simulink model "platoon1"  (R2023a)
settings: Solver=ode2  StartTime=0.0  StopTime=20  FixedStep=1/600  RelTol=1e-3  EnableMultiTasking=on
undefined symbols (not defined in the file or in its folder): HIL, qc_get_step_size
libraries: simulink x29, quarc_library x29, slpidlib x27, cstblocks x23, eeStairGenerator x1
(part 1 of 4)
settings Model: ExtModeTrigDuration=10000  Creator=ritvi  LastModifiedBy=ritvi
settings SolverCC: AlgebraicLoopSolver=TrustRegion  PositivePriorityOrder=on
settings DataIOCC: ReturnWorkspaceOutputs=off
settings DebuggingCC: UnconnectedInputMsg=warning  UnconnectedOutputMsg=warning  UnconnectedLineMsg=warning  ArithmeticOperatorsInVariantConditions=warning
settings HardwareCC: ProdBitPerLong=64  ProdLargestAtomicInteger=LongLong  ProdLargestAtomicFloat=Double  ProdLongLongMode=on  ProdHWDeviceType=ARM Compatible->ARM 64-bit (LP64)
settings ModelReferenceCC: EnableRefExpFcnMdlSchedulingChecks=on
settings SFSimCC: SimUseLocalCustomCode=off  CustomCodeUndefinedFunction=UseInterfaceOnly
settings RTWCC: Description=QUARC Linux Nvidia Target (QCar) Using Toolchain  SystemTargetFile=quarc_linux_nvidia.tlc  TemplateMakefile=quarc_default_tmf  RTWUseLocalCustomCode=off  Toolchain=QUARC linux_nvidia | gmake (64-bit Windows)  BuildConfiguration=Faster Runs
settings CodeAppCC: StateflowObjectComments=on
settings STFCustomTargetCC: SystemTargetFile=quarc_linux_nvidia.tlc
settings GRTTargetCC: ParMdlRefBuildCompliant=off  CompOptLevelCompliant=off  CombineOutputUpdateFcns=off  MatFileLogging=off  CPPClassGenCompliant=off  GRTInterface=on  ExtMode=on  ExtModeMexFile=quarc_comm  ExtModeMexArgs='-w -d /tmp -uri %u', 'tcpip://192.168.1.9'
settings ConfigComp: CovMetricSettings=dswe

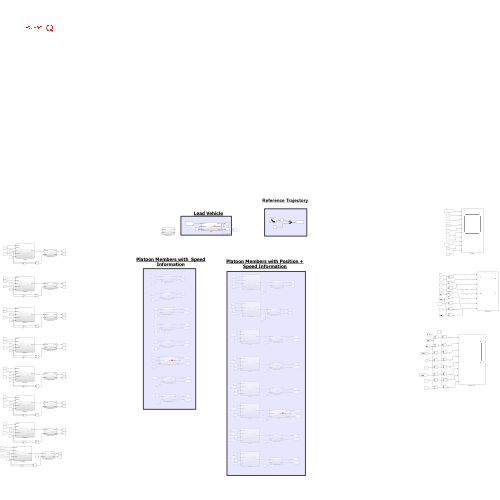
[thumbnail: Simulink's stored preview of the top-level diagram]
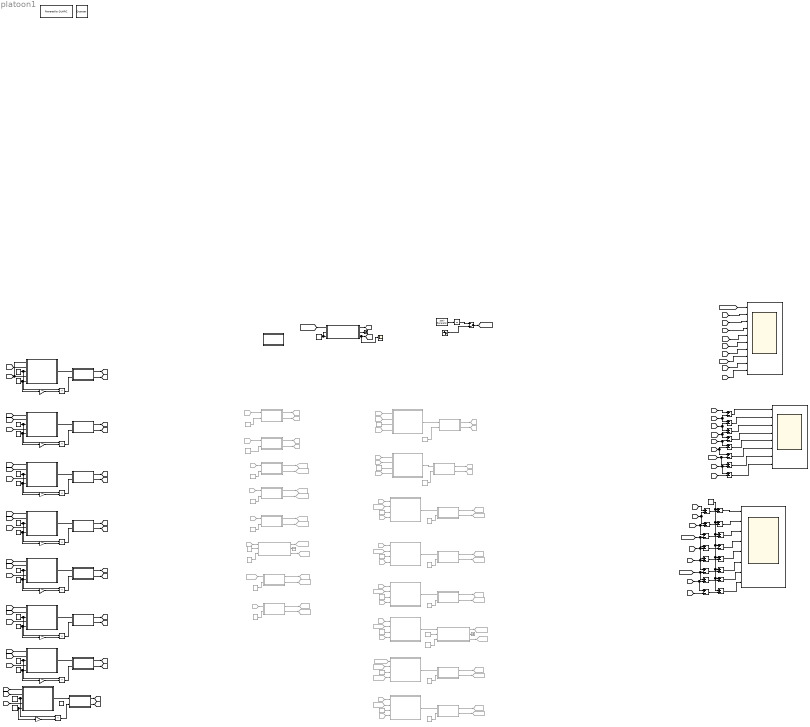
== system platoon1 ==
  note: Platoon Members with Speed Information
  note: Lead Vehicle
  note: Reference Trajectory
  note: Platoon Members with Position + Speed Information
  Add{,1..23} (24 alike) : Sum  Inputs=+-
  Constant : Constant  Value=0
  Constant1 : Constant  Commented=on  Value=0
  Constant{3,6..7,9..10,12,15,18} (8 alike) : Constant  Commented=on  Value=0.5
  Constant11 : Constant  Commented=on  Value=-3.5
  Constant13 : Constant  Commented=on  Value=-4
  Constant{14,19,23,26,28,30,36,40,43} (9 alike) : Constant  Value=0.5
  Constant16 : Constant  Commented=on  Value=-0.5
  Constant17 : Constant
  Constant2 : Constant  Commented=on  Value=-2
  Constant20 : Constant  Commented=on  Value=-1
  Constant21 : Constant  Value=2
  Constant22 : Constant  Commented=on  Value=0
  Constant24 : Constant  Value=3
  Constant25 : Constant  Commented=on  Value=-3.5
  Constant27 : Constant  Value=4
  Constant29 : Constant  Commented=on  Value=-4
  Constant31 : Constant  Value=5
  Constant32 : Constant  Commented=on  Value=-0.5
  Constant33 : Constant  Value=6
  Constant34 : Constant  Commented=on  Value=-2
  Constant35 : Constant  Commented=on  Value=-1
  Constant37 : Constant  Commented=on  Value=-2.5
  Constant38 : Constant  Commented=on  Value=-3
  Constant39 : Constant  Value=7
  Constant4 : Constant  Commented=on  Value=-2.5
  Constant41 : Constant  Commented=on  Value=-1.5
  Constant42 : Constant  Value=8
  Constant44 : Constant  Value=0
  Constant5 : Constant  Commented=on  Value=-3
  Constant8 : Constant  Commented=on  Value=-1.5
  Controller : Subsystem  Commented=on
  Controller1 : Subsystem  Commented=on
  Controller10 : Subsystem
  Controller11 : Subsystem
  Controller12 : Subsystem
  Controller13 : Subsystem
  Controller14 : Subsystem
  Controller15 : Subsystem
  Controller2 : Subsystem  Commented=on
  Controller3 : Subsystem  Commented=on
  Controller4 : Subsystem  Commented=on
  Controller5 : Subsystem  Commented=on
  Controller6 : Subsystem  Commented=on
  Controller7 : Subsystem  Commented=on
  Controller8 : Subsystem
  Controller9 : Subsystem
  Distance errors : Scope  NumInputPorts=8
  From : From  Commented=on  GotoTag=pos1
  From1 : From  Commented=on  GotoTag=pos0
  From10 : From  Commented=on  GotoTag=pos5
  From11 : From  Commented=on  GotoTag=vel4
  From12 : From  Commented=on  GotoTag=pos4
  From13 : From  Commented=on  GotoTag=pos7
  From2 : From  Commented=on  GotoTag=pos2
  From23 : From  Commented=on  GotoTag=vel0
  From24 : From  Commented=on  GotoTag=vel1
  From27 : From  Commented=on  GotoTag=vel6_QCar
  From28 : From  Commented=on  GotoTag=pos6_QCar
  From3 : From  Commented=on  GotoTag=pos1
  From4 : From  Commented=on  GotoTag=pos6_QCar
  From41 : From  Commented=on  GotoTag=pos8
  From42 : From  Commented=on  GotoTag=vel7
  From43 : From  Commented=on  GotoTag=pos7
  From47 : From  Commented=on  GotoTag=pos4
  From48 : From  Commented=on  GotoTag=vel3
  From49 : From  Commented=on  GotoTag=pos3
  From5 : From  Commented=on  GotoTag=vel5
  From6 : From  Commented=on  GotoTag=pos5
  From60 : From  Commented=on  GotoTag=vel4
  From66 : From  Commented=on  GotoTag=vel0
  From68 : From  Commented=on  GotoTag=vel1
  From69 : From  Commented=on  GotoTag=vel6_QCar
  From7 : From  Commented=on  GotoTag=pos3
  From74 : From  Commented=on  GotoTag=vel7
  From77 : From  Commented=on  GotoTag=vel3
  From79 : From  Commented=on  GotoTag=vel5
  From8 : From  Commented=on  GotoTag=vel2
  From82 : From  Commented=on  GotoTag=vel2
  From9 : From  Commented=on  GotoTag=pos2
  Gain{1..8} (8 alike) : Gain  Gain=-1
  Goto10 : Goto  Commented=on  GotoTag=vel2
  Goto11 : Goto  Commented=on  GotoTag=vel6_QCar
  Goto12 : Goto  Commented=on  GotoTag=pos5
  Goto13 : Goto  Commented=on  GotoTag=vel7
  Goto14 : Goto  Commented=on  GotoTag=pos7
  Goto15 : Goto  Commented=on  GotoTag=vel8
  Goto16 : Goto  Commented=on  GotoTag=pos8
  Goto2 : Goto  Commented=on  GotoTag=vel3
  Goto3 : Goto  Commented=on  GotoTag=pos1
  Goto31 : Goto  Commented=on  GotoTag=vel1
  Goto33 : Goto  Commented=on  GotoTag=vel2
  Goto34 : Goto  Commented=on  GotoTag=vel6_QCar
  Goto35 : Goto  Commented=on  GotoTag=pos5
  Goto36 : Goto  Commented=on  GotoTag=vel7
  Goto37 : Goto  Commented=on  GotoTag=pos7
  Goto38 : Goto  Commented=on  GotoTag=vel8
  Goto39 : Goto  Commented=on  GotoTag=pos8
  Goto4 : Goto  Commented=on  GotoTag=pos6_QCar
  Goto40 : Goto  Commented=on  GotoTag=vel3
  Goto41 : Goto  Commented=on  GotoTag=pos1
  Goto42 : Goto  Commented=on  GotoTag=vel1
  Goto43 : Goto  Commented=on  GotoTag=pos6_QCar
  Goto44 : Goto  Commented=on  GotoTag=pos2
  Goto45 : Goto  Commented=on  GotoTag=pos3
  Goto46 : Goto  Commented=on  GotoTag=vel4
  Goto47 : Goto  Commented=on  GotoTag=pos4
  Goto48 : Goto  Commented=on  GotoTag=vel5
  Goto5 : Goto  Commented=on  GotoTag=pos2
  Goto6 : Goto  Commented=on  GotoTag=pos3
  Goto7 : Goto  Commented=on  GotoTag=vel4
  Goto8 : Goto  Commented=on  GotoTag=pos4
  Goto9 : Goto  Commented=on  GotoTag=vel5
  Integrator2 : Integrator
  Manual Switch : ManualSwitch  CurrentSetting=0
  Powered by QUARC : quarc_library/Logos/Powered by QUARC
  Product{,1..7} (8 alike) : Product
  QCar1 : Subsystem  Commented=on
  QCar2 : Subsystem  Commented=on
  QCar4 : Subsystem
  Quanser : quarc_library/Logos/Quanser
  Scope : Scope
  Sine Wave : Sin  Amplitude=0.4  Frequency=0.5  SampleTime=qc_get_step_size
  Stair Generator : eeStairGenerator/Stair Generator  LabelModeActiveChoice=Discrete  TimeInput=[5 7 9 13 15 17]  AmplitudeInput=[0.1 0.15 0 -0.1 -0.15 0]  SampleTime=1/600  RepeatPattern=off  OutDataTypeStr=double
      settings: LibrarySourceBlock=ee_sl_lib/General Control/Stair Generator
  Terminator : Terminator
  Terminator1 : Terminator  Commented=on
  Terminator2 : Terminator  Commented=on
  Velocities : Scope  NumInputPorts=10
  Velocity errors : Scope  NumInputPorts=8
  Virtual Car (TF) : Subsystem
  Virtual Car (TF)1 : Subsystem  Commented=on
  Virtual Car (TF)10 : Subsystem
  Virtual Car (TF)11 : Subsystem
  Virtual Car (TF)12 : Subsystem
  Virtual Car (TF)13 : Subsystem
  Virtual Car (TF)14 : Subsystem
  Virtual Car (TF)15 : Subsystem
  Virtual Car (TF)16 : Subsystem  Commented=on
  Virtual Car (TF)17 : Subsystem  Commented=on
  Virtual Car (TF)18 : Subsystem  Commented=on
  Virtual Car (TF)19 : Subsystem  Commented=on
  Virtual Car (TF)2 : Subsystem  Commented=on
  Virtual Car (TF)20 : Subsystem  Commented=on
  Virtual Car (TF)21 : Subsystem  Commented=on
  Virtual Car (TF)22 : Subsystem
  Virtual Car (TF)3 : Subsystem  Commented=on
  Virtual Car (TF)4 : Subsystem  Commented=on
  Virtual Car (TF)5 : Subsystem  Commented=on
  Virtual Car (TF)6 : Subsystem  Commented=on
  Virtual Car (TF)7 : Subsystem  Commented=on
  Virtual Car (TF)8 : Subsystem  Commented=on
  Virtual Car (TF)9 : Subsystem
  wires:
  QCar1/1(ActSpeed) -> Goto11/1  "v6_Q"
  QCar1/2(ActHeading) -> Terminator1/1
  QCar1/3(position) -> Goto4/1  "p6_Q"
  Controller2/1(Speed) -> QCar1/1(RefSpeed)
  Constant1/1 -> QCar1/2(RefHeading)
  Constant5/1 -> QCar1/3(InitPos)
  From6/1 -> Controller2/1(PosLead)
  From4/1 -> Controller2/2(PosEgo)
  Constant6/1 -> Controller2/3(d_ref)
  From5/1 -> Controller2/4(VelLead)
  Virtual Car (TF)4/1(position) -> Goto8/1  "p4"
  From47/1 -> Controller4/2(PosEgo)
  Add13/1 -> Distance errors/6  "de6"
  Controller1/1(Speed) -> Virtual Car (TF)2/1(RefSpeed)
  Constant8/1 -> Virtual Car (TF)3/2(InitPos)
  [pos1] -> Add18/1, Add6/2
  Controller3/1(Speed) -> Virtual Car (TF)3/1(RefSpeed)
  Constant16/1 -> Virtual Car (TF)1/2(InitPos)
  Virtual Car (TF)1/1(position) -> Goto3/1  "p1"
  Add8/1 -> Add9/2
  [vel3] -> Add2/2, Add3/1
  Add2/1 -> Velocity errors/3  "ve3"
  [vel5] -> Velocities/7
  Virtual Car (TF)3/2(speed) -> Goto2/1  "v3"
  Virtual Car (TF)2/2(speed) -> Goto10/1  "v2"
  Constant20/1 -> Virtual Car (TF)2/2(InitPos)
  QCar4/3(position) -> Scope/1, [pos0]  "p0"
  Virtual Car (TF)1/2(speed) -> Goto31/1  "v1"
  Virtual Car (TF)2/1(position) -> Goto5/1  "p2"
  [vel0] -> Add/1
  [vel0] -> Velocities/2
  [vel1] -> Add/2, Add1/1
  From24/1 -> Controller1/4(VelLead)
  Add3/1 -> Velocity errors/4  "ve4"
  Add6/1 -> Add7/2
  Add5/1 -> Velocity errors/5  "ve5"
  [pos4] -> Add10/1, Add8/2
  Controller/1(Speed) -> Virtual Car (TF)1/1(RefSpeed)
  QCar4/1(ActSpeed) -> [vel0]  "v0"
  Add17/1 -> Distance errors/3  "de3"
  Add1/1 -> Velocity errors/2  "ve2"
  Add16/1 -> Add17/2
  [pos0] -> Add6/1
  Add/1 -> Velocity errors/1  "ve1"
  [pos5] -> Add12/1, Add10/2
  Constant14/1 -> Add7/1, Add19/1, Add17/1, Add9/1, Add11/1, Add23/1, Add20/1, Add13/1
  Add12/1 -> Add13/2
  Add19/1 -> Distance errors/2  "de2"
  Add9/1 -> Distance errors/4  "de4"
  [pos6] -> Add15/1, Add12/2
  Constant2/1 -> Virtual Car (TF)4/2(InitPos)
  Constant3/1 -> Controller4/3(d_ref)
  From48/1 -> Controller4/4(VelLead)
  From13/1 -> Controller6/2(PosEgo)
  From11/1 -> Controller5/4(VelLead)
  [vel6] -> Add14/1, Add4/2
  Controller4/1(Speed) -> Virtual Car (TF)4/1(RefSpeed)
  Constant18/1 -> Controller/3(d_ref)
  Add14/1 -> Velocity errors/7  "ve7"
  From28/1 -> Controller6/1(PosLead)
  Add20/1 -> Distance errors/7  "de7"
  [pos7] -> Add22/1, Add15/2
  From8/1 -> Controller3/4(VelLead)
  Add4/1 -> Velocity errors/6  "ve6"
  [LeadRefSpeed] -> QCar4/1(RefSpeed)
  Controller5/1(Speed) -> Virtual Car (TF)5/1(RefSpeed)
  Virtual Car (TF)3/1(position) -> Goto6/1  "p3"
  Controller6/1(Speed) -> Virtual Car (TF)6/1(RefSpeed)
  From42/1 -> Controller7/4(VelLead)
  Virtual Car (TF)4/2(speed) -> Goto7/1  "v4"
  [vel4] -> Velocities/6
  Virtual Car (TF)6/1(position) -> Goto14/1  "p7"
  Constant4/1 -> Virtual Car (TF)5/2(InitPos)
  [vel7] -> Velocities/9
  Controller7/1(Speed) -> Virtual Car (TF)7/1(RefSpeed)
  From3/1 -> Controller1/1(PosLead)
  [vel2] -> Velocities/4
  [vel3] -> Velocities/5
  From27/1 -> Controller6/4(VelLead)
  From12/1 -> Controller5/1(PosLead)
  Add18/1 -> Add19/2
  Virtual Car (TF)6/2(speed) -> Goto13/1  "v7"
  Virtual Car (TF)5/2(speed) -> Goto9/1  "v5"
  [vel2] -> Add1/2, Add2/1
  From/1 -> Controller/2(PosEgo)
  [pos3] -> Add8/1, Add16/2
  [LeadRefSpeed] -> Velocities/1
  From10/1 -> Controller5/2(PosEgo)
  [vel6] -> Velocities/8
  Constant7/1 -> Controller5/3(d_ref)
  Constant15/1 -> Controller7/3(d_ref)
  Constant/1 -> QCar4/2(RefHeading), QCar4/3(InitPos)
  Add11/1 -> Distance errors/5  "de5"
  From41/1 -> Controller7/2(PosEgo)
  From2/1 -> Controller1/2(PosEgo)
  From9/1 -> Controller3/1(PosLead)
  Constant11/1 -> Virtual Car (TF)6/2(InitPos)
  Add10/1 -> Add11/2
  From7/1 -> Controller3/2(PosEgo)
  Constant9/1 -> Controller3/3(d_ref)
  Add7/1 -> Distance errors/1  "de1"
  Constant12/1 -> Controller6/3(d_ref)
  Virtual Car (TF)7/1(position) -> Goto16/1  "p8"
  [vel1] -> Velocities/3
  [vel5] -> Add4/1, Add5/2
  Constant13/1 -> Virtual Car (TF)7/2(InitPos)
  [vel4] -> Add3/2, Add5/1
  From1/1 -> Controller/1(PosLead)
  Virtual Car (TF)5/1(position) -> Goto12/1  "p5"
  Virtual Car (TF)7/2(speed) -> Goto15/1  "v8"
  [pos2] -> Add16/1, Add18/2
  [vel7] -> Add21/1, Add14/2
  Constant10/1 -> Controller1/3(d_ref)
  From43/1 -> Controller7/1(PosLead)
  Add15/1 -> Add20/2
  From49/1 -> Controller4/1(PosLead)
  From23/1 -> Controller/4(VelLead)
  [vel8] -> Velocities/10
  [vel8] -> Add21/2
  Add21/1 -> Velocity errors/8  "ve8"
  Add22/1 -> Add23/2
  [pos8] -> Add22/2
  Add23/1 -> Distance errors/8  "de8"
  Virtual Car (TF)19/1(position) -> Goto35/1  "p5"
  Virtual Car (TF)21/2(speed) -> Goto38/1  "v8"
  From69/1 -> Virtual Car (TF)20/1(RefSpeed)
  Virtual Car (TF)19/2(speed) -> Goto48/1  "v5"
  Virtual Car (TF)20/2(speed) -> Goto36/1  "v7"
  Virtual Car (TF)17/1(position) -> Goto45/1  "p3"
  Virtual Car (TF)18/2(speed) -> Goto46/1  "v4"
  From74/1 -> Virtual Car (TF)21/1(RefSpeed)
  From82/1 -> Virtual Car (TF)17/1(RefSpeed)
  Virtual Car (TF)20/1(position) -> Goto37/1  "p7"
  From60/1 -> Virtual Car (TF)19/1(RefSpeed)
  Constant34/1 -> Virtual Car (TF)18/2(InitPos)
  Virtual Car (TF)16/1(position) -> Goto44/1  "p2"
  Constant35/1 -> Virtual Car (TF)16/2(InitPos)
  Virtual Car (TF)21/1(position) -> Goto39/1  "p8"
  Virtual Car (TF)17/2(speed) -> Goto40/1  "v3"
  Virtual Car (TF)16/2(speed) -> Goto33/1  "v2"
  Constant32/1 -> Virtual Car (TF)8/2(InitPos)
  Constant37/1 -> Virtual Car (TF)19/2(InitPos)
  Constant25/1 -> Virtual Car (TF)20/2(InitPos)
  Virtual Car (TF)8/1(position) -> Goto41/1  "p1"
  Constant41/1 -> Virtual Car (TF)17/2(InitPos)
  From66/1 -> Virtual Car (TF)8/1(RefSpeed)
  Virtual Car (TF)18/1(position) -> Goto47/1  "p4"
  From77/1 -> Virtual Car (TF)18/1(RefSpeed)
  Virtual Car (TF)8/2(speed) -> Goto42/1  "v1"
  From79/1 -> QCar2/1(RefSpeed)
  Constant29/1 -> Virtual Car (TF)21/2(InitPos)
  QCar2/2(ActHeading) -> Terminator2/1
  QCar2/1(ActSpeed) -> Goto34/1  "v6_Q"
  Constant38/1 -> QCar2/3(InitPos)
  QCar2/3(position) -> Goto43/1  "p6_Q"
  Constant22/1 -> QCar2/2(RefHeading)
  From68/1 -> Virtual Car (TF)16/1(RefSpeed)
  [pos0] -> Controller13/4(PosLead)
  Virtual Car (TF)14/1(position) -> [pos7]  "p7"
  Product6/1 -> Virtual Car (TF)14/2(InitPos)
  Gain7/1 -> Product6/2
  Controller13/1(Speed) -> Virtual Car (TF)14/1(RefSpeed)
  [pos6] -> Controller13/1(PosPred)
  Constant40/1 -> Product6/1, Controller13/3(d_ref)
  Constant39/1 -> Controller13/5(i), Gain7/1
  [pos4] -> Controller11/1(PosPred)
  Constant31/1 -> Controller11/5(i), Gain5/1
  Virtual Car (TF)12/2(speed) -> [vel5]  "v5"
  Constant30/1 -> Product4/1, Controller11/3(d_ref)
  [pos0] -> Controller11/4(PosLead)
  Gain5/1 -> Product4/2
  Product4/1 -> Virtual Car (TF)12/2(InitPos)
  [pos5] -> Controller11/2(PosEgo)
  Controller11/1(Speed) -> Virtual Car (TF)12/1(RefSpeed)
  Constant33/1 -> Controller12/5(i), Gain6/1
  Gain6/1 -> Product5/2
  [pos6] -> Controller12/2(PosEgo)
  Controller12/1(Speed) -> Virtual Car (TF)13/1(RefSpeed)
  Virtual Car (TF)13/1(position) -> [pos6]  "p6"
  Product1/1 -> Virtual Car (TF)9/2(InitPos)
  [pos2] -> Controller9/2(PosEgo)
  Virtual Car (TF)9/1(position) -> [pos2]  "p2"
  Controller9/1(Speed) -> Virtual Car (TF)9/1(RefSpeed)
  Constant23/1 -> Product1/1, Controller9/3(d_ref)
  [pos0] -> Controller9/4(PosLead)
  Virtual Car (TF)14/2(speed) -> [vel7]  "v7"
  [pos1] -> Controller8/2(PosEgo)
  [pos7] -> Controller13/2(PosEgo)
  [pos0] -> Controller8/1(PosPred), Controller8/4(PosLead)
  [pos5] -> Controller12/1(PosPred)
  Constant28/1 -> Product3/1, Controller10/3(d_ref)
  Virtual Car (TF)11/2(speed) -> [vel4]  "v4"
  Gain2/1 -> Product1/2
  [pos0] -> Controller10/4(PosLead)
  Constant27/1 -> Controller10/5(i), Gain4/1
  Product3/1 -> Virtual Car (TF)11/2(InitPos)
  Virtual Car (TF)15/2(speed) -> [vel1]  "v1"
  [pos0] -> Controller12/4(PosLead)
  Gain4/1 -> Product3/2
  Gain1/1 -> Product/2
  [pos3] -> Controller10/1(PosPred)
  Constant19/1 -> Product/1, Controller8/3(d_ref)
  Product5/1 -> Virtual Car (TF)13/2(InitPos)
  Controller8/1(Speed) -> Virtual Car (TF)15/1(RefSpeed)
  Virtual Car (TF)15/1(position) -> [pos1]  "p1"
  Virtual Car (TF)12/1(position) -> [pos5]  "p5"
  Constant26/1 -> Product2/1, Controller14/3(d_ref)
  Virtual Car (TF)10/2(speed) -> [vel3]  "v3"
  [pos0] -> Controller14/4(PosLead)
  Constant24/1 -> Controller14/5(i), Gain3/1
  [pos2] -> Controller14/1(PosPred)
  Virtual Car (TF)13/2(speed) -> [vel6]  "v6"
  Constant21/1 -> Controller9/5(i), Gain2/1
  Gain3/1 -> Product2/2
  Constant36/1 -> Product5/1, Controller12/3(d_ref)
  Product2/1 -> Virtual Car (TF)10/2(InitPos)
  Virtual Car (TF)10/1(position) -> [pos3]  "p3"
  Constant17/1 -> Controller8/5(i), Gain1/1
  Controller10/1(Speed) -> Virtual Car (TF)11/1(RefSpeed)
  Controller14/1(Speed) -> Virtual Car (TF)10/1(RefSpeed)
  Virtual Car (TF)11/1(position) -> [pos4]  "p4"
  [pos1] -> Controller9/1(PosPred)
  [pos4] -> Controller10/2(PosEgo)
  Virtual Car (TF)9/2(speed) -> [vel2]  "v2"
  [pos3] -> Controller14/2(PosEgo)
  Product/1 -> Virtual Car (TF)15/2(InitPos)
  [pos8] -> Controller15/2(PosEgo)
  [pos0] -> Controller15/4(PosLead)
  Product7/1 -> Virtual Car (TF)22/2(InitPos)
  Controller15/1(Speed) -> Virtual Car (TF)22/1(RefSpeed)
  Constant42/1 -> Controller15/5(i), Gain8/1
  Gain8/1 -> Product7/2
  Constant43/1 -> Product7/1, Controller15/3(d_ref)
  [pos7] -> Controller15/1(PosPred)
  Virtual Car (TF)22/2(speed) -> [vel8]  "v8"
  Virtual Car (TF)22/1(position) -> [pos8]  "p8"
  Integrator2/1 -> Manual Switch/1
  Stair Generator/1 -> Integrator2/1
  Sine Wave/1 -> Manual Switch/2
  Manual Switch/1 -> [LeadRefSpeed]  "v_ref"
  QCar4/2(ActHeading) -> Terminator/1

== system platoon1/Controller ==
  PosLead : Inport
  PosEgo : Inport  Port=2
  d_ref : Inport  Port=3
  VelLead : Inport  Port=4
  Add : Sum  Inputs=+-
  Add1 : Sum  Inputs=+-
  Add2 : Sum  Inputs=+-
  Discrete Derivative : simulink/Discrete/Discrete Derivative  Commented=on  gainval=1.0  ICPrevScaledInput=0.0  OutMin=[]  OutMax=[]  OutDataType=fixdt(1, 16)  OutScaling=2^-10  DoSatur=off
  Integrator : Integrator  Commented=on
  Kd : Gain  Commented=on
  Ki : Gain  Commented=on
  Kp : Gain  Commented=on
  PID Controller : slpidlib/PID Controller  Controller=PID  Form=Parallel  TimeDomain=Continuous-time  UseExternalTs=off  SampleTime=-1  IntegratorMethod=Forward Euler  FilterMethod=Forward Euler  ControllerParametersSource=internal  P=3.40490772994016  I=1.59625421797035  UseKiTs=off  D=0.569076840427193  N=614.736952919996  UseFilter=on  TunerSelectOption=Transfer Function Based (PID Tuner App)  InitialConditionSource=internal  InitialConditionForIntegrator=0  InitialConditionForFilter=0  DifferentiatorICPrevScaledInput=0  ExternalReset=none  TrackingMode=off  Kt=1  LimitOutput=off  SatLimitsSource=internal  UpperSaturationLimit=inf  LowerSaturationLimit=-inf  LinearizeAsGain=on  AntiWindupMode=none  Kb=1  LimitIntegrator=off  UpperIntegratorSaturationLimit=inf  LowerIntegratorSaturationLimit=-inf  POutMin=[]  POutMax=[]  IOutMin=[]  IOutMax=[]  DOutMin=[]  DOutMax=[]  NOutMin=[]  NOutMax=[]  SumOutMin=[]  SumOutMax=[]  SaturationOutMin=[]  SaturationOutMax=[]  PParamMin=[]  PParamMax=[]  IParamMin=[]  IParamMax=[]  DParamMin=[]  DParamMax=[]  NParamMin=[]  NParamMax=[]  KbParamMin=[]  KbParamMax=[]  KtParamMin=[]  KtParamMax=[]  KbOutMin=[]  KbOutMax=[]  KtOutMin=[]  KtOutMax=[]  IntegratorOutMin=[]  IntegratorOutMax=[]  FilterOutMin=[]  FilterOutMax=[]  SumI1OutMin=[]  SumI1OutMax=[]  SumI2OutMin=[]  SumI2OutMax=[]  SumI3OutMin=[]  SumI3OutMax=[]  SumI4OutMin=[]  SumI4OutMax=[]  SumDOutMin=[]  SumDOutMax=[]  DifferentiatorOutMin=[]  DifferentiatorOutMax=[]  FilterDiffOutCoefMin=[]  FilterDiffOutCoefMax=[]  ReciprocalOutMin=[]  ReciprocalOutMax=[]  SumDenOutMin=[]  SumDenOutMax=[]  SumNumOutMin=[]  SumNumOutMax=[]  DivideOutMin=[]  DivideOutMax=[]  UdiffTsProdOutMin=[]  UdiffTsProdOutMax=[]  NTsProdOutMin=[]  NTsProdOutMax=[]  UintegralTsProdOutMin=[]  UintegralTsProdOutMax=[]  UngainTsProdOutMin=[]  UngainTsProdOutMax=[]  ClampingZeroOutDataTypeStr=Inherit: Inherit via back propagation  ClampingZeroOutMin=[]  ClampingZeroOutMax=[]  FilterDenConstantOutDataTypeStr=Inherit: Inherit via back propagation  FilterDenConstantOutMin=[]  FilterDenConstantOutMax=[]  PCopyOutDataTypeStr=Inherit: Inherit via back propagation  PCopyOutMin=[]  PCopyOutMax=[]  NCopyOutDataTypeStr=Inherit: Inherit via back propagation  NCopyOutMin=[]  NCopyOutMax=[]  IntegratorContinuousStateAttributes=''  IntegratorStateMustResolveToSignalObject=off  IntegratorRTWStateStorageClass=Auto  FilterContinuousStateAttributes=''  FilterStateMustResolveToSignalObject=off  FilterRTWStateStorageClass=Auto  ParallelPVariant=InternalParameters  IdealPVariant=Disabled  IVariant=InternalParameters  DVariant=InternalParameters  IntegratorVariant=Continuous  SatVariant=Disabled  AWVariant=Passthrough  PCopyVariant=Disabled  TRVariant=Disabled  FdbkBlocksVariant=Forward  IdealPFdbkVariant=Disabled  SatFdbkVariant=Disabled  DerivativeFilterVariant=ContFilter  NVariant=InternalParameters  NCopyVariant=Disabled  FilterICVariant=InternalICsFilter  IntegratorICVariant=InternalICs  ExternalResetVariant=Disabled  TRSumVariant=Passthrough  SumFdbkVariant=Disabled  SumVariant=Sum_PID  TsampFilterVariant=InternalTs  TsampNgainVariant=Passthrough  TsampIntegralVariant=Disabled_SignalSpec  ExternalSaturationOutDataTypeStr=Inherit: Same as second input
  Sum : Sum  Commented=on  Inputs=+++
  Speed : Outport
  wires:
  PosLead/1 -> Add/1
  PosEgo/1 -> Add/2
  Add/1 -> Add1/2  "d_act"
  d_ref/1 -> Add1/1
  Add1/1 -> PID Controller/1  "d_error"
  Kd/1 -> Discrete Derivative/1
  Ki/1 -> Integrator/1
  Kp/1 -> Sum/1
  Integrator/1 -> Sum/2
  Discrete Derivative/1 -> Sum/3
  VelLead/1 -> Add2/1
  Add2/1 -> Speed/1
  PID Controller/1 -> Add2/2

== system platoon1/Controller1 ==
  PosLead : Inport
  PosEgo : Inport  Port=2
  d_ref : Inport  Port=3
  VelLead : Inport  Port=4
  Add : Sum  Inputs=+-
  Add1 : Sum  Inputs=+-
  Add2 : Sum  Inputs=+-
  Discrete Derivative : simulink/Discrete/Discrete Derivative  Commented=on  gainval=1.0  ICPrevScaledInput=0.0  OutMin=[]  OutMax=[]  OutDataType=fixdt(1, 16)  OutScaling=2^-10  DoSatur=off
  Integrator : Integrator  Commented=on
  Kd : Gain  Commented=on
  Ki : Gain  Commented=on
  Kp : Gain  Commented=on
  PID Controller : slpidlib/PID Controller  Controller=PID  Form=Parallel  TimeDomain=Continuous-time  UseExternalTs=off  SampleTime=-1  IntegratorMethod=Forward Euler  FilterMethod=Forward Euler  ControllerParametersSource=internal  P=3.40490772994016  I=1.59625421797035  UseKiTs=off  D=0.569076840427193  N=614.736952919996  UseFilter=on  TunerSelectOption=Transfer Function Based (PID Tuner App)  InitialConditionSource=internal  InitialConditionForIntegrator=0  InitialConditionForFilter=0  DifferentiatorICPrevScaledInput=0  ExternalReset=none  TrackingMode=off  Kt=1  LimitOutput=off  SatLimitsSource=internal  UpperSaturationLimit=inf  LowerSaturationLimit=-inf  LinearizeAsGain=on  AntiWindupMode=none  Kb=1  LimitIntegrator=off  UpperIntegratorSaturationLimit=inf  LowerIntegratorSaturationLimit=-inf  POutMin=[]  POutMax=[]  IOutMin=[]  IOutMax=[]  DOutMin=[]  DOutMax=[]  NOutMin=[]  NOutMax=[]  SumOutMin=[]  SumOutMax=[]  SaturationOutMin=[]  SaturationOutMax=[]  PParamMin=[]  PParamMax=[]  IParamMin=[]  IParamMax=[]  DParamMin=[]  DParamMax=[]  NParamMin=[]  NParamMax=[]  KbParamMin=[]  KbParamMax=[]  KtParamMin=[]  KtParamMax=[]  KbOutMin=[]  KbOutMax=[]  KtOutMin=[]  KtOutMax=[]  IntegratorOutMin=[]  IntegratorOutMax=[]  FilterOutMin=[]  FilterOutMax=[]  SumI1OutMin=[]  SumI1OutMax=[]  SumI2OutMin=[]  SumI2OutMax=[]  SumI3OutMin=[]  SumI3OutMax=[]  SumI4OutMin=[]  SumI4OutMax=[]  SumDOutMin=[]  SumDOutMax=[]  DifferentiatorOutMin=[]  DifferentiatorOutMax=[]  FilterDiffOutCoefMin=[]  FilterDiffOutCoefMax=[]  ReciprocalOutMin=[]  ReciprocalOutMax=[]  SumDenOutMin=[]  SumDenOutMax=[]  SumNumOutMin=[]  SumNumOutMax=[]  DivideOutMin=[]  DivideOutMax=[]  UdiffTsProdOutMin=[]  UdiffTsProdOutMax=[]  NTsProdOutMin=[]  NTsProdOutMax=[]  UintegralTsProdOutMin=[]  UintegralTsProdOutMax=[]  UngainTsProdOutMin=[]  UngainTsProdOutMax=[]  ClampingZeroOutDataTypeStr=Inherit: Inherit via back propagation  ClampingZeroOutMin=[]  ClampingZeroOutMax=[]  FilterDenConstantOutDataTypeStr=Inherit: Inherit via back propagation  FilterDenConstantOutMin=[]  FilterDenConstantOutMax=[]  PCopyOutDataTypeStr=Inherit: Inherit via back propagation  PCopyOutMin=[]  PCopyOutMax=[]  NCopyOutDataTypeStr=Inherit: Inherit via back propagation  NCopyOutMin=[]  NCopyOutMax=[]  IntegratorContinuousStateAttributes=''  IntegratorStateMustResolveToSignalObject=off  IntegratorRTWStateStorageClass=Auto  FilterContinuousStateAttributes=''  FilterStateMustResolveToSignalObject=off  FilterRTWStateStorageClass=Auto  ParallelPVariant=InternalParameters  IdealPVariant=Disabled  IVariant=InternalParameters  DVariant=InternalParameters  IntegratorVariant=Continuous  SatVariant=Disabled  AWVariant=Passthrough  PCopyVariant=Disabled  TRVariant=Disabled  FdbkBlocksVariant=Forward  IdealPFdbkVariant=Disabled  SatFdbkVariant=Disabled  DerivativeFilterVariant=ContFilter  NVariant=InternalParameters  NCopyVariant=Disabled  FilterICVariant=InternalICsFilter  IntegratorICVariant=InternalICs  ExternalResetVariant=Disabled  TRSumVariant=Passthrough  SumFdbkVariant=Disabled  SumVariant=Sum_PID  TsampFilterVariant=InternalTs  TsampNgainVariant=Passthrough  TsampIntegralVariant=Disabled_SignalSpec  ExternalSaturationOutDataTypeStr=Inherit: Same as second input
  Sum : Sum  Commented=on  Inputs=+++
  Speed : Outport
  wires:
  PosLead/1 -> Add/1
  PosEgo/1 -> Add/2
  Add/1 -> Add1/2  "d_act"
  d_ref/1 -> Add1/1
  Kd/1 -> Discrete Derivative/1
  Ki/1 -> Integrator/1
  Kp/1 -> Sum/1
  Integrator/1 -> Sum/2
  Discrete Derivative/1 -> Sum/3
  VelLead/1 -> Add2/1
  Add2/1 -> Speed/1
  Add1/1 -> PID Controller/1  "d_error"
  PID Controller/1 -> Add2/2

== system platoon1/Controller10 ==
  PosPred : Inport
  PosEgo : Inport  Port=2
  d_ref : Inport  Port=3
  PosLead : Inport  Port=4
  i : Inport  Port=5
  Add : Sum  Inputs=+-
  Add1 : Sum  Inputs=-+
  Add2 : Sum
  Add3 : Sum  Inputs=+-
  Add4 : Sum  Inputs=-+
  Integrator : Integrator
  PID Controller : slpidlib/PID Controller  Controller=PID  Form=Parallel  TimeDomain=Continuous-time  UseExternalTs=off  SampleTime=-1  IntegratorMethod=Forward Euler  FilterMethod=Forward Euler  ControllerParametersSource=internal  P=0.33095280227445  I=0.0676054764431606  UseKiTs=off  D=0.347839718693587  N=40.6182647095365  UseFilter=on  TunerSelectOption=Transfer Function Based (PID Tuner App)  InitialConditionSource=internal  InitialConditionForIntegrator=0  InitialConditionForFilter=0  DifferentiatorICPrevScaledInput=0  ExternalReset=none  TrackingMode=off  Kt=1  LimitOutput=off  SatLimitsSource=internal  UpperSaturationLimit=inf  LowerSaturationLimit=-inf  LinearizeAsGain=on  AntiWindupMode=none  Kb=1  LimitIntegrator=off  UpperIntegratorSaturationLimit=inf  LowerIntegratorSaturationLimit=-inf  POutMin=[]  POutMax=[]  IOutMin=[]  IOutMax=[]  DOutMin=[]  DOutMax=[]  NOutMin=[]  NOutMax=[]  SumOutMin=[]  SumOutMax=[]  SaturationOutMin=[]  SaturationOutMax=[]  PParamMin=[]  PParamMax=[]  IParamMin=[]  IParamMax=[]  DParamMin=[]  DParamMax=[]  NParamMin=[]  NParamMax=[]  KbParamMin=[]  KbParamMax=[]  KtParamMin=[]  KtParamMax=[]  KbOutMin=[]  KbOutMax=[]  KtOutMin=[]  KtOutMax=[]  IntegratorOutMin=[]  IntegratorOutMax=[]  FilterOutMin=[]  FilterOutMax=[]  SumI1OutMin=[]  SumI1OutMax=[]  SumI2OutMin=[]  SumI2OutMax=[]  SumI3OutMin=[]  SumI3OutMax=[]  SumI4OutMin=[]  SumI4OutMax=[]  SumDOutMin=[]  SumDOutMax=[]  DifferentiatorOutMin=[]  DifferentiatorOutMax=[]  FilterDiffOutCoefMin=[]  FilterDiffOutCoefMax=[]  ReciprocalOutMin=[]  ReciprocalOutMax=[]  SumDenOutMin=[]  SumDenOutMax=[]  SumNumOutMin=[]  SumNumOutMax=[]  DivideOutMin=[]  DivideOutMax=[]  UdiffTsProdOutMin=[]  UdiffTsProdOutMax=[]  NTsProdOutMin=[]  NTsProdOutMax=[]  UintegralTsProdOutMin=[]  UintegralTsProdOutMax=[]  UngainTsProdOutMin=[]  UngainTsProdOutMax=[]  ClampingZeroOutDataTypeStr=Inherit: Inherit via back propagation  ClampingZeroOutMin=[]  ClampingZeroOutMax=[]  FilterDenConstantOutDataTypeStr=Inherit: Inherit via back propagation  FilterDenConstantOutMin=[]  FilterDenConstantOutMax=[]  PCopyOutDataTypeStr=Inherit: Inherit via back propagation  PCopyOutMin=[]  PCopyOutMax=[]  NCopyOutDataTypeStr=Inherit: Inherit via back propagation  NCopyOutMin=[]  NCopyOutMax=[]  IntegratorContinuousStateAttributes=''  IntegratorStateMustResolveToSignalObject=off  IntegratorRTWStateStorageClass=Auto  FilterContinuousStateAttributes=''  FilterStateMustResolveToSignalObject=off  FilterRTWStateStorageClass=Auto  ParallelPVariant=InternalParameters  IdealPVariant=Disabled  IVariant=InternalParameters  DVariant=InternalParameters  IntegratorVariant=Continuous  SatVariant=Disabled  AWVariant=Passthrough  PCopyVariant=Disabled  TRVariant=Disabled  FdbkBlocksVariant=Forward  IdealPFdbkVariant=Disabled  SatFdbkVariant=Disabled  DerivativeFilterVariant=ContFilter  NVariant=InternalParameters  NCopyVariant=Disabled  FilterICVariant=InternalICsFilter  IntegratorICVariant=InternalICs  ExternalResetVariant=Disabled  TRSumVariant=Passthrough  SumFdbkVariant=Disabled  SumVariant=Sum_PID  TsampFilterVariant=InternalTs  TsampNgainVariant=Passthrough  TsampIntegralVariant=Disabled_SignalSpec  ExternalSaturationOutDataTypeStr=Inherit: Same as second input
  PID Controller1 : slpidlib/PID Controller  Controller=PID  Form=Parallel  TimeDomain=Continuous-time  UseExternalTs=off  SampleTime=-1  IntegratorMethod=Forward Euler  FilterMethod=Forward Euler  ControllerParametersSource=internal  P=0.0689075408458366  I=0.00109879069900871  UseKiTs=off  D=0.960150912828831  N=312.36902011058  UseFilter=on  TunerSelectOption=Transfer Function Based (PID Tuner App)  InitialConditionSource=internal  InitialConditionForIntegrator=0  InitialConditionForFilter=0  DifferentiatorICPrevScaledInput=0  ExternalReset=none  TrackingMode=off  Kt=1  LimitOutput=off  SatLimitsSource=internal  UpperSaturationLimit=inf  LowerSaturationLimit=-inf  LinearizeAsGain=on  AntiWindupMode=none  Kb=1  LimitIntegrator=off  UpperIntegratorSaturationLimit=inf  LowerIntegratorSaturationLimit=-inf  POutMin=[]  POutMax=[]  IOutMin=[]  IOutMax=[]  DOutMin=[]  DOutMax=[]  NOutMin=[]  NOutMax=[]  SumOutMin=[]  SumOutMax=[]  SaturationOutMin=[]  SaturationOutMax=[]  PParamMin=[]  PParamMax=[]  IParamMin=[]  IParamMax=[]  DParamMin=[]  DParamMax=[]  NParamMin=[]  NParamMax=[]  KbParamMin=[]  KbParamMax=[]  KtParamMin=[]  KtParamMax=[]  KbOutMin=[]  KbOutMax=[]  KtOutMin=[]  KtOutMax=[]  IntegratorOutMin=[]  IntegratorOutMax=[]  FilterOutMin=[]  FilterOutMax=[]  SumI1OutMin=[]  SumI1OutMax=[]  SumI2OutMin=[]  SumI2OutMax=[]  SumI3OutMin=[]  SumI3OutMax=[]  SumI4OutMin=[]  SumI4OutMax=[]  SumDOutMin=[]  SumDOutMax=[]  DifferentiatorOutMin=[]  DifferentiatorOutMax=[]  FilterDiffOutCoefMin=[]  FilterDiffOutCoefMax=[]  ReciprocalOutMin=[]  ReciprocalOutMax=[]  SumDenOutMin=[]  SumDenOutMax=[]  SumNumOutMin=[]  SumNumOutMax=[]  DivideOutMin=[]  DivideOutMax=[]  UdiffTsProdOutMin=[]  UdiffTsProdOutMax=[]  NTsProdOutMin=[]  NTsProdOutMax=[]  UintegralTsProdOutMin=[]  UintegralTsProdOutMax=[]  UngainTsProdOutMin=[]  UngainTsProdOutMax=[]  ClampingZeroOutDataTypeStr=Inherit: Inherit via back propagation  ClampingZeroOutMin=[]  ClampingZeroOutMax=[]  FilterDenConstantOutDataTypeStr=Inherit: Inherit via back propagation  FilterDenConstantOutMin=[]  FilterDenConstantOutMax=[]  PCopyOutDataTypeStr=Inherit: Inherit via back propagation  PCopyOutMin=[]  PCopyOutMax=[]  NCopyOutDataTypeStr=Inherit: Inherit via back propagation  NCopyOutMin=[]  NCopyOutMax=[]  IntegratorContinuousStateAttributes=''  IntegratorStateMustResolveToSignalObject=off  IntegratorRTWStateStorageClass=Auto  FilterContinuousStateAttributes=''  FilterStateMustResolveToSignalObject=off  FilterRTWStateStorageClass=Auto  ParallelPVariant=InternalParameters  IdealPVariant=Disabled  IVariant=InternalParameters  DVariant=InternalParameters  IntegratorVariant=Continuous  SatVariant=Disabled  AWVariant=Passthrough  PCopyVariant=Disabled  TRVariant=Disabled  FdbkBlocksVariant=Forward  IdealPFdbkVariant=Disabled  SatFdbkVariant=Disabled  DerivativeFilterVariant=ContFilter  NVariant=InternalParameters  NCopyVariant=Disabled  FilterICVariant=InternalICsFilter  IntegratorICVariant=InternalICs  ExternalResetVariant=Disabled  TRSumVariant=Passthrough  SumFdbkVariant=Disabled  SumVariant=Sum_PID  TsampFilterVariant=InternalTs  TsampNgainVariant=Passthrough  TsampIntegralVariant=Disabled_SignalSpec  ExternalSaturationOutDataTypeStr=Inherit: Same as second input
  Product : Product
  Speed : Outport
  wires:
  PosPred/1 -> Add/1
  PosEgo/1 -> Add/2, Add3/2
  Add/1 -> Add1/2  "d_act"
  d_ref/1 -> Product/2, Add1/1
  Add1/1 -> PID Controller/1  "d_error_pred"
  Add2/1 -> Integrator/1
  PID Controller/1 -> Add2/2
  PosLead/1 -> Add3/1
  Add3/1 -> Add4/2  "d_act"
  Product/1 -> Add4/1
  i/1 -> Product/1
  Add4/1 -> PID Controller1/1  "d_error_lead"
  PID Controller1/1 -> Add2/1
  Integrator/1 -> Speed/1

== system platoon1/Controller11 ==
  PosPred : Inport
  PosEgo : Inport  Port=2
  d_ref : Inport  Port=3
  PosLead : Inport  Port=4
  i : Inport  Port=5
  Add : Sum  Inputs=+-
  Add1 : Sum  Inputs=-+
  Add2 : Sum
  Add3 : Sum  Inputs=+-
  Add4 : Sum  Inputs=-+
  Integrator : Integrator
  PID Controller : slpidlib/PID Controller  Controller=PID  Form=Parallel  TimeDomain=Continuous-time  UseExternalTs=off  SampleTime=-1  IntegratorMethod=Forward Euler  FilterMethod=Forward Euler  ControllerParametersSource=internal  P=0.33095280227445  I=0.0676054764431606  UseKiTs=off  D=0.347839718693587  N=40.6182647095365  UseFilter=on  TunerSelectOption=Transfer Function Based (PID Tuner App)  InitialConditionSource=internal  InitialConditionForIntegrator=0  InitialConditionForFilter=0  DifferentiatorICPrevScaledInput=0  ExternalReset=none  TrackingMode=off  Kt=1  LimitOutput=off  SatLimitsSource=internal  UpperSaturationLimit=inf  LowerSaturationLimit=-inf  LinearizeAsGain=on  AntiWindupMode=none  Kb=1  LimitIntegrator=off  UpperIntegratorSaturationLimit=inf  LowerIntegratorSaturationLimit=-inf  POutMin=[]  POutMax=[]  IOutMin=[]  IOutMax=[]  DOutMin=[]  DOutMax=[]  NOutMin=[]  NOutMax=[]  SumOutMin=[]  SumOutMax=[]  SaturationOutMin=[]  SaturationOutMax=[]  PParamMin=[]  PParamMax=[]  IParamMin=[]  IParamMax=[]  DParamMin=[]  DParamMax=[]  NParamMin=[]  NParamMax=[]  KbParamMin=[]  KbParamMax=[]  KtParamMin=[]  KtParamMax=[]  KbOutMin=[]  KbOutMax=[]  KtOutMin=[]  KtOutMax=[]  IntegratorOutMin=[]  IntegratorOutMax=[]  FilterOutMin=[]  FilterOutMax=[]  SumI1OutMin=[]  SumI1OutMax=[]  SumI2OutMin=[]  SumI2OutMax=[]  SumI3OutMin=[]  SumI3OutMax=[]  SumI4OutMin=[]  SumI4OutMax=[]  SumDOutMin=[]  SumDOutMax=[]  DifferentiatorOutMin=[]  DifferentiatorOutMax=[]  FilterDiffOutCoefMin=[]  FilterDiffOutCoefMax=[]  ReciprocalOutMin=[]  ReciprocalOutMax=[]  SumDenOutMin=[]  SumDenOutMax=[]  SumNumOutMin=[]  SumNumOutMax=[]  DivideOutMin=[]  DivideOutMax=[]  UdiffTsProdOutMin=[]  UdiffTsProdOutMax=[]  NTsProdOutMin=[]  NTsProdOutMax=[]  UintegralTsProdOutMin=[]  UintegralTsProdOutMax=[]  UngainTsProdOutMin=[]  UngainTsProdOutMax=[]  ClampingZeroOutDataTypeStr=Inherit: Inherit via back propagation  ClampingZeroOutMin=[]  ClampingZeroOutMax=[]  FilterDenConstantOutDataTypeStr=Inherit: Inherit via back propagation  FilterDenConstantOutMin=[]  FilterDenConstantOutMax=[]  PCopyOutDataTypeStr=Inherit: Inherit via back propagation  PCopyOutMin=[]  PCopyOutMax=[]  NCopyOutDataTypeStr=Inherit: Inherit via back propagation  NCopyOutMin=[]  NCopyOutMax=[]  IntegratorContinuousStateAttributes=''  IntegratorStateMustResolveToSignalObject=off  IntegratorRTWStateStorageClass=Auto  FilterContinuousStateAttributes=''  FilterStateMustResolveToSignalObject=off  FilterRTWStateStorageClass=Auto  ParallelPVariant=InternalParameters  IdealPVariant=Disabled  IVariant=InternalParameters  DVariant=InternalParameters  IntegratorVariant=Continuous  SatVariant=Disabled  AWVariant=Passthrough  PCopyVariant=Disabled  TRVariant=Disabled  FdbkBlocksVariant=Forward  IdealPFdbkVariant=Disabled  SatFdbkVariant=Disabled  DerivativeFilterVariant=ContFilter  NVariant=InternalParameters  NCopyVariant=Disabled  FilterICVariant=InternalICsFilter  IntegratorICVariant=InternalICs  ExternalResetVariant=Disabled  TRSumVariant=Passthrough  SumFdbkVariant=Disabled  SumVariant=Sum_PID  TsampFilterVariant=InternalTs  TsampNgainVariant=Passthrough  TsampIntegralVariant=Disabled_SignalSpec  ExternalSaturationOutDataTypeStr=Inherit: Same as second input
  PID Controller1 : slpidlib/PID Controller  Controller=PID  Form=Parallel  TimeDomain=Continuous-time  UseExternalTs=off  SampleTime=-1  IntegratorMethod=Forward Euler  FilterMethod=Forward Euler  ControllerParametersSource=internal  P=0.0689075408458366  I=0.00109879069900871  UseKiTs=off  D=0.960150912828831  N=312.36902011058  UseFilter=on  TunerSelectOption=Transfer Function Based (PID Tuner App)  InitialConditionSource=internal  InitialConditionForIntegrator=0  InitialConditionForFilter=0  DifferentiatorICPrevScaledInput=0  ExternalReset=none  TrackingMode=off  Kt=1  LimitOutput=off  SatLimitsSource=internal  UpperSaturationLimit=inf  LowerSaturationLimit=-inf  LinearizeAsGain=on  AntiWindupMode=none  Kb=1  LimitIntegrator=off  UpperIntegratorSaturationLimit=inf  LowerIntegratorSaturationLimit=-inf  POutMin=[]  POutMax=[]  IOutMin=[]  IOutMax=[]  DOutMin=[]  DOutMax=[]  NOutMin=[]  NOutMax=[]  SumOutMin=[]  SumOutMax=[]  SaturationOutMin=[]  SaturationOutMax=[]  PParamMin=[]  PParamMax=[]  IParamMin=[]  IParamMax=[]  DParamMin=[]  DParamMax=[]  NParamMin=[]  NParamMax=[]  KbParamMin=[]  KbParamMax=[]  KtParamMin=[]  KtParamMax=[]  KbOutMin=[]  KbOutMax=[]  KtOutMin=[]  KtOutMax=[]  IntegratorOutMin=[]  IntegratorOutMax=[]  FilterOutMin=[]  FilterOutMax=[]  SumI1OutMin=[]  SumI1OutMax=[]  SumI2OutMin=[]  SumI2OutMax=[]  SumI3OutMin=[]  SumI3OutMax=[]  SumI4OutMin=[]  SumI4OutMax=[]  SumDOutMin=[]  SumDOutMax=[]  DifferentiatorOutMin=[]  DifferentiatorOutMax=[]  FilterDiffOutCoefMin=[]  FilterDiffOutCoefMax=[]  ReciprocalOutMin=[]  ReciprocalOutMax=[]  SumDenOutMin=[]  SumDenOutMax=[]  SumNumOutMin=[]  SumNumOutMax=[]  DivideOutMin=[]  DivideOutMax=[]  UdiffTsProdOutMin=[]  UdiffTsProdOutMax=[]  NTsProdOutMin=[]  NTsProdOutMax=[]  UintegralTsProdOutMin=[]  UintegralTsProdOutMax=[]  UngainTsProdOutMin=[]  UngainTsProdOutMax=[]  ClampingZeroOutDataTypeStr=Inherit: Inherit via back propagation  ClampingZeroOutMin=[]  ClampingZeroOutMax=[]  FilterDenConstantOutDataTypeStr=Inherit: Inherit via back propagation  FilterDenConstantOutMin=[]  FilterDenConstantOutMax=[]  PCopyOutDataTypeStr=Inherit: Inherit via back propagation  PCopyOutMin=[]  PCopyOutMax=[]  NCopyOutDataTypeStr=Inherit: Inherit via back propagation  NCopyOutMin=[]  NCopyOutMax=[]  IntegratorContinuousStateAttributes=''  IntegratorStateMustResolveToSignalObject=off  IntegratorRTWStateStorageClass=Auto  FilterContinuousStateAttributes=''  FilterStateMustResolveToSignalObject=off  FilterRTWStateStorageClass=Auto  ParallelPVariant=InternalParameters  IdealPVariant=Disabled  IVariant=InternalParameters  DVariant=InternalParameters  IntegratorVariant=Continuous  SatVariant=Disabled  AWVariant=Passthrough  PCopyVariant=Disabled  TRVariant=Disabled  FdbkBlocksVariant=Forward  IdealPFdbkVariant=Disabled  SatFdbkVariant=Disabled  DerivativeFilterVariant=ContFilter  NVariant=InternalParameters  NCopyVariant=Disabled  FilterICVariant=InternalICsFilter  IntegratorICVariant=InternalICs  ExternalResetVariant=Disabled  TRSumVariant=Passthrough  SumFdbkVariant=Disabled  SumVariant=Sum_PID  TsampFilterVariant=InternalTs  TsampNgainVariant=Passthrough  TsampIntegralVariant=Disabled_SignalSpec  ExternalSaturationOutDataTypeStr=Inherit: Same as second input
  Product : Product
  Speed : Outport
  wires:
  PosPred/1 -> Add/1
  PosEgo/1 -> Add/2, Add3/2
  Add/1 -> Add1/2  "d_act"
  d_ref/1 -> Product/2, Add1/1
  Add1/1 -> PID Controller/1  "d_error_pred"
  Add2/1 -> Integrator/1
  PID Controller/1 -> Add2/2
  PosLead/1 -> Add3/1
  Add3/1 -> Add4/2  "d_act"
  Product/1 -> Add4/1
  i/1 -> Product/1
  Add4/1 -> PID Controller1/1  "d_error_lead"
  PID Controller1/1 -> Add2/1
  Integrator/1 -> Speed/1

== system platoon1/Controller12 ==
  PosPred : Inport
  PosEgo : Inport  Port=2
  d_ref : Inport  Port=3
  PosLead : Inport  Port=4
  i : Inport  Port=5
  Add : Sum  Inputs=+-
  Add1 : Sum  Inputs=-+
  Add2 : Sum
  Add3 : Sum  Inputs=+-
  Add4 : Sum  Inputs=-+
  Integrator : Integrator
  PID Controller : slpidlib/PID Controller  Controller=PID  Form=Parallel  TimeDomain=Continuous-time  UseExternalTs=off  SampleTime=-1  IntegratorMethod=Forward Euler  FilterMethod=Forward Euler  ControllerParametersSource=internal  P=0.33095280227445  I=0.0676054764431606  UseKiTs=off  D=0.347839718693587  N=40.6182647095365  UseFilter=on  TunerSelectOption=Transfer Function Based (PID Tuner App)  InitialConditionSource=internal  InitialConditionForIntegrator=0  InitialConditionForFilter=0  DifferentiatorICPrevScaledInput=0  ExternalReset=none  TrackingMode=off  Kt=1  LimitOutput=off  SatLimitsSource=internal  UpperSaturationLimit=inf  LowerSaturationLimit=-inf  LinearizeAsGain=on  AntiWindupMode=none  Kb=1  LimitIntegrator=off  UpperIntegratorSaturationLimit=inf  LowerIntegratorSaturationLimit=-inf  POutMin=[]  POutMax=[]  IOutMin=[]  IOutMax=[]  DOutMin=[]  DOutMax=[]  NOutMin=[]  NOutMax=[]  SumOutMin=[]  SumOutMax=[]  SaturationOutMin=[]  SaturationOutMax=[]  PParamMin=[]  PParamMax=[]  IParamMin=[]  IParamMax=[]  DParamMin=[]  DParamMax=[]  NParamMin=[]  NParamMax=[]  KbParamMin=[]  KbParamMax=[]  KtParamMin=[]  KtParamMax=[]  KbOutMin=[]  KbOutMax=[]  KtOutMin=[]  KtOutMax=[]  IntegratorOutMin=[]  IntegratorOutMax=[]  FilterOutMin=[]  FilterOutMax=[]  SumI1OutMin=[]  SumI1OutMax=[]  SumI2OutMin=[]  SumI2OutMax=[]  SumI3OutMin=[]  SumI3OutMax=[]  SumI4OutMin=[]  SumI4OutMax=[]  SumDOutMin=[]  SumDOutMax=[]  DifferentiatorOutMin=[]  DifferentiatorOutMax=[]  FilterDiffOutCoefMin=[]  FilterDiffOutCoefMax=[]  ReciprocalOutMin=[]  ReciprocalOutMax=[]  SumDenOutMin=[]  SumDenOutMax=[]  SumNumOutMin=[]  SumNumOutMax=[]  DivideOutMin=[]  DivideOutMax=[]  UdiffTsProdOutMin=[]  UdiffTsProdOutMax=[]  NTsProdOutMin=[]  NTsProdOutMax=[]  UintegralTsProdOutMin=[]  UintegralTsProdOutMax=[]  UngainTsProdOutMin=[]  UngainTsProdOutMax=[]  ClampingZeroOutDataTypeStr=Inherit: Inherit via back propagation  ClampingZeroOutMin=[]  ClampingZeroOutMax=[]  FilterDenConstantOutDataTypeStr=Inherit: Inherit via back propagation  FilterDenConstantOutMin=[]  FilterDenConstantOutMax=[]  PCopyOutDataTypeStr=Inherit: Inherit via back propagation  PCopyOutMin=[]  PCopyOutMax=[]  NCopyOutDataTypeStr=Inherit: Inherit via back propagation  NCopyOutMin=[]  NCopyOutMax=[]  IntegratorContinuousStateAttributes=''  IntegratorStateMustResolveToSignalObject=off  IntegratorRTWStateStorageClass=Auto  FilterContinuousStateAttributes=''  FilterStateMustResolveToSignalObject=off  FilterRTWStateStorageClass=Auto  ParallelPVariant=InternalParameters  IdealPVariant=Disabled  IVariant=InternalParameters  DVariant=InternalParameters  IntegratorVariant=Continuous  SatVariant=Disabled  AWVariant=Passthrough  PCopyVariant=Disabled  TRVariant=Disabled  FdbkBlocksVariant=Forward  IdealPFdbkVariant=Disabled  SatFdbkVariant=Disabled  DerivativeFilterVariant=ContFilter  NVariant=InternalParameters  NCopyVariant=Disabled  FilterICVariant=InternalICsFilter  IntegratorICVariant=InternalICs  ExternalResetVariant=Disabled  TRSumVariant=Passthrough  SumFdbkVariant=Disabled  SumVariant=Sum_PID  TsampFilterVariant=InternalTs  TsampNgainVariant=Passthrough  TsampIntegralVariant=Disabled_SignalSpec  ExternalSaturationOutDataTypeStr=Inherit: Same as second input
  PID Controller1 : slpidlib/PID Controller  Controller=PID  Form=Parallel  TimeDomain=Continuous-time  UseExternalTs=off  SampleTime=-1  IntegratorMethod=Forward Euler  FilterMethod=Forward Euler  ControllerParametersSource=internal  P=0.0689075408458366  I=0.00109879069900871  UseKiTs=off  D=0.960150912828831  N=312.36902011058  UseFilter=on  TunerSelectOption=Transfer Function Based (PID Tuner App)  InitialConditionSource=internal  InitialConditionForIntegrator=0  InitialConditionForFilter=0  DifferentiatorICPrevScaledInput=0  ExternalReset=none  TrackingMode=off  Kt=1  LimitOutput=off  SatLimitsSource=internal  UpperSaturationLimit=inf  LowerSaturationLimit=-inf  LinearizeAsGain=on  AntiWindupMode=none  Kb=1  LimitIntegrator=off  UpperIntegratorSaturationLimit=inf  LowerIntegratorSaturationLimit=-inf  POutMin=[]  POutMax=[]  IOutMin=[]  IOutMax=[]  DOutMin=[]  DOutMax=[]  NOutMin=[]  NOutMax=[]  SumOutMin=[]  SumOutMax=[]  SaturationOutMin=[]  SaturationOutMax=[]  PParamMin=[]  PParamMax=[]  IParamMin=[]  IParamMax=[]  DParamMin=[]  DParamMax=[]  NParamMin=[]  NParamMax=[]  KbParamMin=[]  KbParamMax=[]  KtParamMin=[]  KtParamMax=[]  KbOutMin=[]  KbOutMax=[]  KtOutMin=[]  KtOutMax=[]  IntegratorOutMin=[]  IntegratorOutMax=[]  FilterOutMin=[]  FilterOutMax=[]  SumI1OutMin=[]  SumI1OutMax=[]  SumI2OutMin=[]  SumI2OutMax=[]  SumI3OutMin=[]  SumI3OutMax=[]  SumI4OutMin=[]  SumI4OutMax=[]  SumDOutMin=[]  SumDOutMax=[]  DifferentiatorOutMin=[]  DifferentiatorOutMax=[]  FilterDiffOutCoefMin=[]  FilterDiffOutCoefMax=[]  ReciprocalOutMin=[]  ReciprocalOutMax=[]  SumDenOutMin=[]  SumDenOutMax=[]  SumNumOutMin=[]  SumNumOutMax=[]  DivideOutMin=[]  DivideOutMax=[]  UdiffTsProdOutMin=[]  UdiffTsProdOutMax=[]  NTsProdOutMin=[]  NTsProdOutMax=[]  UintegralTsProdOutMin=[]  UintegralTsProdOutMax=[]  UngainTsProdOutMin=[]  UngainTsProdOutMax=[]  ClampingZeroOutDataTypeStr=Inherit: Inherit via back propagation  ClampingZeroOutMin=[]  ClampingZeroOutMax=[]  FilterDenConstantOutDataTypeStr=Inherit: Inherit via back propagation  FilterDenConstantOutMin=[]  FilterDenConstantOutMax=[]  PCopyOutDataTypeStr=Inherit: Inherit via back propagation  PCopyOutMin=[]  PCopyOutMax=[]  NCopyOutDataTypeStr=Inherit: Inherit via back propagation  NCopyOutMin=[]  NCopyOutMax=[]  IntegratorContinuousStateAttributes=''  IntegratorStateMustResolveToSignalObject=off  IntegratorRTWStateStorageClass=Auto  FilterContinuousStateAttributes=''  FilterStateMustResolveToSignalObject=off  FilterRTWStateStorageClass=Auto  ParallelPVariant=InternalParameters  IdealPVariant=Disabled  IVariant=InternalParameters  DVariant=InternalParameters  IntegratorVariant=Continuous  SatVariant=Disabled  AWVariant=Passthrough  PCopyVariant=Disabled  TRVariant=Disabled  FdbkBlocksVariant=Forward  IdealPFdbkVariant=Disabled  SatFdbkVariant=Disabled  DerivativeFilterVariant=ContFilter  NVariant=InternalParameters  NCopyVariant=Disabled  FilterICVariant=InternalICsFilter  IntegratorICVariant=InternalICs  ExternalResetVariant=Disabled  TRSumVariant=Passthrough  SumFdbkVariant=Disabled  SumVariant=Sum_PID  TsampFilterVariant=InternalTs  TsampNgainVariant=Passthrough  TsampIntegralVariant=Disabled_SignalSpec  ExternalSaturationOutDataTypeStr=Inherit: Same as second input
  Product : Product
  Speed : Outport
  wires:
  PosPred/1 -> Add/1
  PosEgo/1 -> Add/2, Add3/2
  Add/1 -> Add1/2  "d_act"
  d_ref/1 -> Product/2, Add1/1
  Add1/1 -> PID Controller/1  "d_error_pred"
  Add2/1 -> Integrator/1
  PID Controller/1 -> Add2/2
  PosLead/1 -> Add3/1
  Add3/1 -> Add4/2  "d_act"
  Product/1 -> Add4/1
  i/1 -> Product/1
  Add4/1 -> PID Controller1/1  "d_error_lead"
  PID Controller1/1 -> Add2/1
  Integrator/1 -> Speed/1
